simulink model "neuropid1_nlin1_2a"  (R2013a)
settings: Solver=ode3  StartTime=0.0  StopTime=cas  FixedStep=Ts  RelTol=1e-3
values from neighbouring files (symbols this model uses):
  k1 = pb(3)    [generacia_neuropid1_2.m]
  k2 = pb(4)    [generacia_neuropid1_2.m]
  r1 = pb(1)    [generacia_neuropid1_2.m]
  r2 = pb(2)    [generacia_neuropid1_2.m]
  Ts = 0.001    [generacia_neuropid1_2.m]
  W2 = ones(1,3)*100000    [generacia_neuropid1_2.m]
undefined symbols (not defined in the file or in its folder): W1
libraries: simulink x3
settings Model: Creator=admin-genetic  LastModifiedBy=admin-genetic

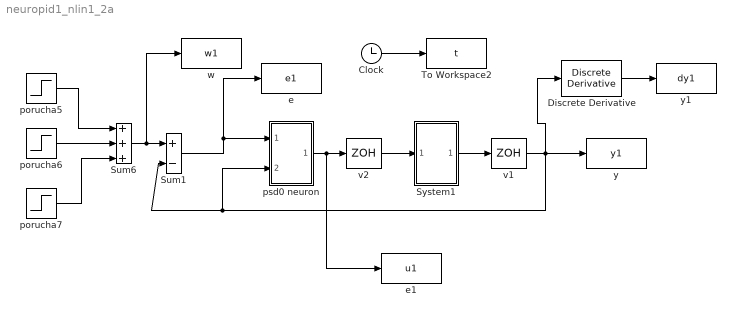
== system neuropid1_nlin1_2a ==
  Clock : Clock
  Discrete Derivative : simulink/Discrete/Discrete Derivative  gainval=1.0  ICPrevScaledInput=0.0  InputProcessing=Inherited  OutMin=[]  OutMax=[]  OutDataType=fixdt(1, 16)  OutScaling=2^-10  DoSatur=off
  Sum1 : Sum  Inputs=+-
  Sum6 : Sum  Inputs=+++
  System1 : Subsystem
  To Workspace2 : ToWorkspace  VariableName=t  SampleTime=-1
  e : ToWorkspace  VariableName=e1  SampleTime=-1
  e1 : ToWorkspace  VariableName=u1  SampleTime=-1
  porucha5 : Step  After=r1  SampleTime=0
  porucha6 : Step  Time=3  After=-r1  SampleTime=0
  porucha7 : Step  Time=6  After=r2  SampleTime=0
  psd0 neuron : Subsystem
  v1 : ZeroOrderHold  SampleTime=Ts
  v2 : ZeroOrderHold  SampleTime=Ts
  w : ToWorkspace  VariableName=w1  SampleTime=-1
  y : ToWorkspace  VariableName=y1  SampleTime=-1
  y1 : ToWorkspace  VariableName=dy1  SampleTime=-1
  wires:
  porucha5/1 -> Sum6/1
  porucha6/1 -> Sum6/2
  porucha7/1 -> Sum6/3
  Clock/1 -> To Workspace2/1
  System1/1(Out1) -> v1/1
  Sum6/1 -> w/1, Sum1/1
  v1/1 -> Discrete Derivative/1, psd0 neuron/2(In2), Sum1/2, y/1
  Sum1/1 -> psd0 neuron/1(In1), e/1
  v2/1 -> System1/1(In1)
  Discrete Derivative/1 -> y1/1
  psd0 neuron/1(Out1) -> e1/1, v2/1

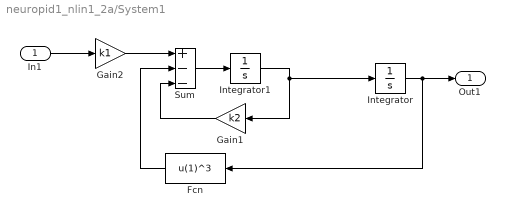
== system neuropid1_nlin1_2a/System1 ==
  In1 : Inport
  Fcn : Fcn  Expr=u(1)^3
  Gain1 : Gain  Gain=k2  SaturateOnIntegerOverflow=on  OutDataTypeStr=Inherit: Same as input  ParamDataTypeStr=Inherit: Same as input
  Gain2 : Gain  Gain=k1  SaturateOnIntegerOverflow=on  OutDataTypeStr=Inherit: Same as input  ParamDataTypeStr=Inherit: Same as input
  Integrator : Integrator
  Integrator1 : Integrator
  Sum : Sum  Inputs=+--  SaturateOnIntegerOverflow=on  InputSameDT=on  OutDataTypeStr=Inherit: Same as first input
  Out1 : Outport
  wires:
  Integrator1/1 -> Integrator/1, Gain1/1
  In1/1 -> Gain2/1
  Gain1/1 -> Sum/3
  Integrator/1 -> Fcn/1, Out1/1
  Fcn/1 -> Sum/2
  Sum/1 -> Integrator1/1
  Gain2/1 -> Sum/1

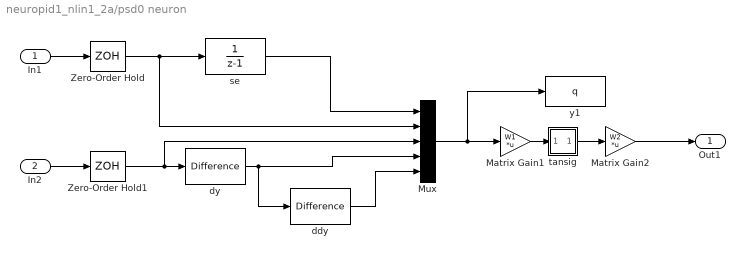
== system neuropid1_nlin1_2a/psd0 neuron ==
  In1 : Inport
  In2 : Inport  Port=2
  Matrix Gain1 : Gain  Gain=W1  Multiplication=Matrix(K*u)  SampleTime=Ts  SaturateOnIntegerOverflow=on  OutDataTypeStr=Inherit: Same as input  ParamDataTypeStr=Inherit: Same as input
  Matrix Gain2 : Gain  Gain=W2  Multiplication=Matrix(K*u)  SampleTime=Ts  SaturateOnIntegerOverflow=on  OutDataTypeStr=Inherit: Same as input  ParamDataTypeStr=Inherit: Same as input
  Mux : Mux  Inputs=5
  Zero-Order Hold : ZeroOrderHold  SampleTime=Ts
  Zero-Order Hold1 : ZeroOrderHold  SampleTime=Ts
  ddy : simulink/Discrete/Difference  ICPrevInput=0.0  OutMin=[]  OutMax=[]  OutDataType=fixdt(1, 16)  OutScaling=2^-10  DoSatur=off
  dy : simulink/Discrete/Difference  ICPrevInput=0.0  OutMin=[]  OutMax=[]  OutDataType=fixdt(1, 16)  OutScaling=2^-10  DoSatur=off
  se : DiscreteTransferFcn  Denominator=[1 -1]  SampleTime=Ts
  tansig : Subsystem
      mask Display: plot([-1 1],[0 0],[-1 -.9 -.8 -.7 -.6 -.5 -.4 -.3 -.2 -.1 0 .1 .2 .3 .4 .5 .6 .7 .8 .9 1],2./(1+exp(-8*[-1 -.9 -.8 -.7 -.6 -.5 -.4 -.3 -.2 -.1 0 .1 .2 .3 .4 .5 .6 .7 .8 .9 1]))-1)
  y1 : ToWorkspace  VariableName=q  SampleTime=-1
  Out1 : Outport
  wires:
  In2/1 -> Zero-Order Hold1/1
  tansig/1(a) -> Matrix Gain2/1
  In1/1 -> Zero-Order Hold/1
  Matrix Gain1/1 -> tansig/1(n)
  Matrix Gain2/1 -> Out1/1
  Mux/1 -> y1/1, Matrix Gain1/1
  Zero-Order Hold/1 -> Mux/2, se/1
  Zero-Order Hold1/1 -> Mux/3, dy/1
  se/1 -> Mux/1
  dy/1 -> ddy/1, Mux/4
  ddy/1 -> Mux/5

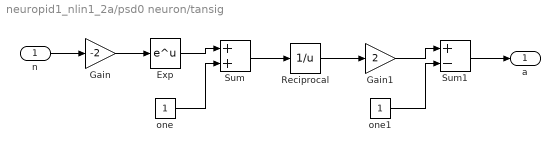
== system neuropid1_nlin1_2a/psd0 neuron/tansig ==
  n : Inport
  Exp : Math  SaturateOnIntegerOverflow=on
  Gain : Gain  Gain=-2  SaturateOnIntegerOverflow=on  OutDataTypeStr=Inherit: Same as input  ParamDataTypeStr=Inherit: Same as input
  Gain1 : Gain  Gain=2  SaturateOnIntegerOverflow=on  OutDataTypeStr=Inherit: Same as input  ParamDataTypeStr=Inherit: Same as input
  Reciprocal : Math  Operator=reciprocal  SaturateOnIntegerOverflow=on
  Sum : Sum  SaturateOnIntegerOverflow=on  InputSameDT=on  OutDataTypeStr=Inherit: Same as first input
  Sum1 : Sum  Inputs=+-  SaturateOnIntegerOverflow=on  InputSameDT=on  OutDataTypeStr=Inherit: Same as first input
  one : Constant
  one1 : Constant
  a : Outport
  wires:
  n/1 -> Gain/1
  Gain/1 -> Exp/1
  Exp/1 -> Sum/1
  one/1 -> Sum/2
  Sum/1 -> Reciprocal/1
  Reciprocal/1 -> Gain1/1
  Gain1/1 -> Sum1/1
  one1/1 -> Sum1/2
  Sum1/1 -> a/1
